simulink model "gNautilus_UDP_8Channels"  (R2017b)
settings: Solver=FixedStepDiscrete  StartTime=0.0  StopTime=inf  RelTol=1e-3  EnableMultiTasking=on
model workspace (MAT data in the model file):
  cfg_native : struct (value not decoded)
  en_add_channels = 127
  host_ip = 2130706433
  host_port = 50223
  local_ip = 2130706433
  local_port = 50224
  num_en_channels = 8
  num_samples = 8
  sample_rate = 500
  serial_number = 'NB-2016.09.84'
undefined symbols (not defined in the file): NB
libraries: gtecHighspeedLib x2, dspnetwork x1, gNautilusLib x1, gNautilusTools x1
settings Model: Creator=g.tec Maresch  LastModifiedBy=Gabriel
settings DataIOCC: LimitDataPoints=on  SaveFormat=Array
settings OptimizationCC: ExpressionDepthLimit=2147483647  LifeSpan=inf
settings DebuggingCC: UnderspecifiedInitializationDetection=Classic  MergeDetectMultiDrivingBlocksExec=none  SolverPrmCheckMsg=warning  FcnCallInpInsideContextMsg=warning  FrameProcessingCompatibilityMsg=none  StateNameClashWarn=warning  SFUnexpectedBacktrackingDiag=warning  SFNoUnconditionalDefaultTransitionDiag=warning  SFExecutionAtInitializationDiag=none
settings HardwareCC: ProdBitPerInt=16  ProdBitPerPointer=16  ProdBitPerSizeT=16  ProdBitPerPtrDiffT=16  ProdLargestAtomicFloat=None  ProdEndianess=Unspecified  ProdWordSize=8  ProdShiftRightIntArith=off  ProdHWDeviceType=Intel->8051 Compatible
settings ModelReferenceCC: PropagateSignalLabelsOutOfModel=off
settings SFSimCC: SFSimEcho=off  SimCtrlC=off  SimIntegrity=off
settings CodeAppCC: StateflowObjectComments=on
settings GRTTargetCC: TargetLangStandard=C89/C90 (ANSI)  GeneratePreprocessorConditionals=Disable all  CombineOutputUpdateFcns=off  GRTInterface=on
settings ConfigComp: CovMetricSettings=dw  CovHtmlReporting=on  CovSaveCumulativeToWorkspaceVar=on  CovSaveSingleToWorkspaceVar=on  CovExternalEMLEnable=off

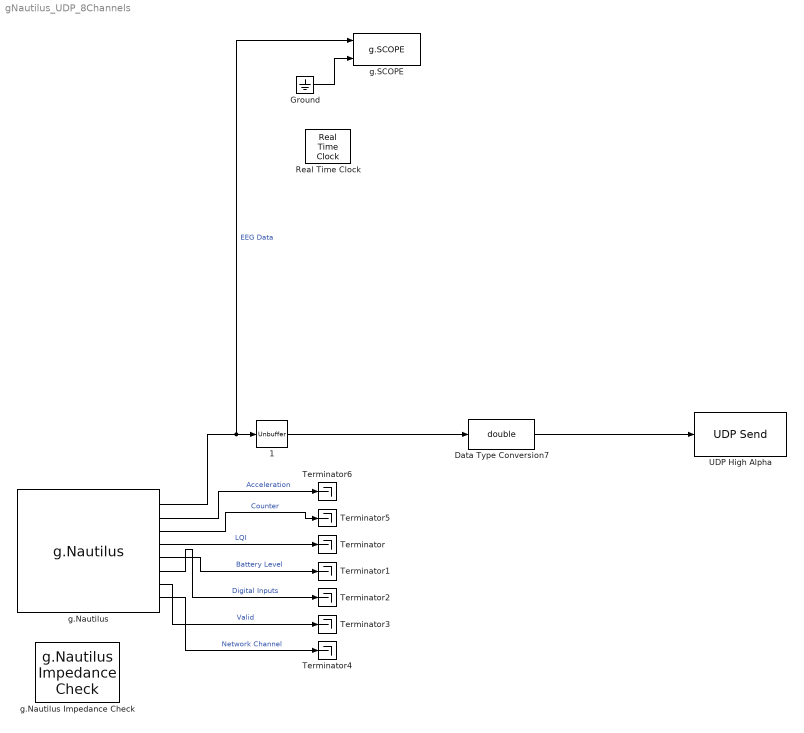
== system gNautilus_UDP_8Channels ==
  1 : Unbuffer
  Data Type Conversion7 : DataTypeConversion  OutDataTypeStr=double
  Ground : Ground
  Real Time Clock : gtecHighspeedLib/Real Time Clock  timeprofile=on
      settings: SourceProductName=g.tec Highspeed Library
  Terminator{,1..6} (7 alike) : Terminator
  UDP High Alpha : dspnetwork/UDP Send  remoteURL='192.168.0.2'  remotePort=12345  localURL='0.0.0.0'  localPortSource=Automatically determine  localPort=-1  sampletime=-1  blockPlatform=[]  separateLengthPort=0
      settings: SourceProductName=DSP System Toolbox  SourceProductBaseCode=DS
  g.Nautilus : gNautilusLib/g.Nautilus  Tag=g.Nautilus  Description=Operates a g.Nautilus device and provides acquired data on its outputs.  sample_rate=500  local_ip=2130706433  local_port=50224  host_ip=2130706433  host_port=50223  serial_number=NB-2016.09.84  num_samples=8  num_en_channels=8  add_channels=127
      settings: SourceProductName=g.Nautilus
  g.Nautilus Impedance Check : gNautilusTools/g.Nautilus Impedance Check
  g.SCOPE : gtecHighspeedLib/g.SCOPE
      settings: SourceProductName=g.tec Highspeed Library
  wires:
  g.Nautilus/1 -> g.SCOPE/1, 1/1  "EEG Data"
  g.Nautilus/8 -> Terminator4/1  "Network Channel"
  g.Nautilus/7 -> Terminator3/1  "Valid"
  g.Nautilus/6 -> Terminator2/1  "Digital Inputs"
  g.Nautilus/5 -> Terminator1/1  "Battery Level"
  g.Nautilus/4 -> Terminator/1  "LQI"
  g.Nautilus/3 -> Terminator5/1  "Counter"
  g.Nautilus/2 -> Terminator6/1  "Acceleration"
  Ground/1 -> g.SCOPE/2
  Data Type Conversion7/1 -> UDP High Alpha/1
  1/1 -> Data Type Conversion7/1
